simulink model "yuanhub_math_fun"  (R2023a)
settings: configuration reference "config" (kept outside this file)
model workspace (MAT data in the model file):
  timer_s = Simulink.Signal
  timer_s.Description = '时间计数器 s'
  timer_s.DataType = 'single'
  timer_s.Dimensions = -1
  timer_s.DimensionsMode = 'auto'
  timer_s.Complexity = 'auto'
  timer_s.SampleTime = -1
  timer_s.SamplingMode = 'auto'
  timer_s.InitialValue = '0'
settings Model: DataDictionary=model_config.sldd  Creator=huangcheng  LastModifiedBy=Administrator
settings ConfigSetRef: SourceName=config

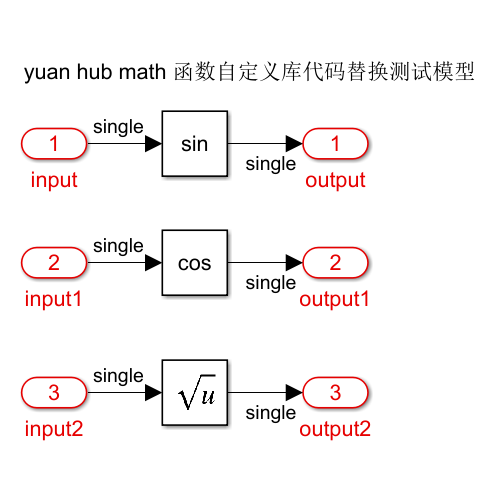
[thumbnail: Simulink's stored preview of the top-level diagram]
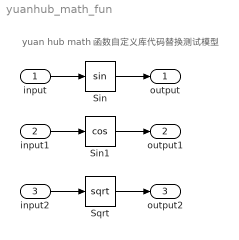
== system yuanhub_math_fun ==
  note: yuan hub math 函数自定义库代码替换测试模型
  input : Inport  OutDataTypeStr=single
  input1 : Inport  Port=2  OutDataTypeStr=single
  input2 : Inport  Port=3  OutDataTypeStr=single
  Sin : Trigonometry
  Sin1 : Trigonometry  Operator=cos
  Sqrt : Sqrt
  output : Outport  OutDataTypeStr=single
  output1 : Outport  Port=2  OutDataTypeStr=single
  output2 : Outport  Port=3  OutDataTypeStr=single
  wires:
  input/1 -> Sin/1
  Sin/1 -> output/1
  Sin1/1 -> output1/1
  input1/1 -> Sin1/1
  input2/1 -> Sqrt/1
  Sqrt/1 -> output2/1
